simulink model "Task5_without_Scalar"  (R2023b)
settings: Solver=FixedStepAuto  StartTime=0.0  StopTime=500  FixedStep=.02  RelTol=1e-3
values from neighbouring files (symbols this model uses):
  A_Long = [Xu                    Xw                        -w0                            -gravity*cos(theta0) ... (first row only)    [Longitudinal_Autopilot.m]
  B_Long = [Xde                         Xdth ... (first row only)    [Longitudinal_Autopilot.m]
  C_Long = eye(4)    [Longitudinal_Autopilot.m]
  D_Long = zeros(4,2)    [Longitudinal_Autopilot.m]
undefined symbols (not defined in the file or in its folder): states_0, theta0, u0, w0
libraries: simulink_extras x7, cstblocks x2
settings Model: Creator=Saif Mohamed  LastModifiedBy=Saif Mohamed

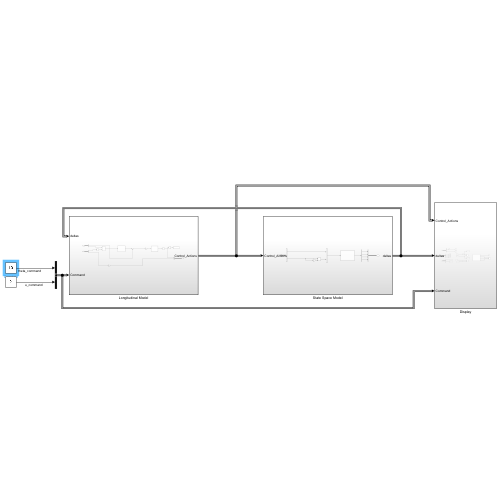
[thumbnail: Simulink's stored preview of the top-level diagram]
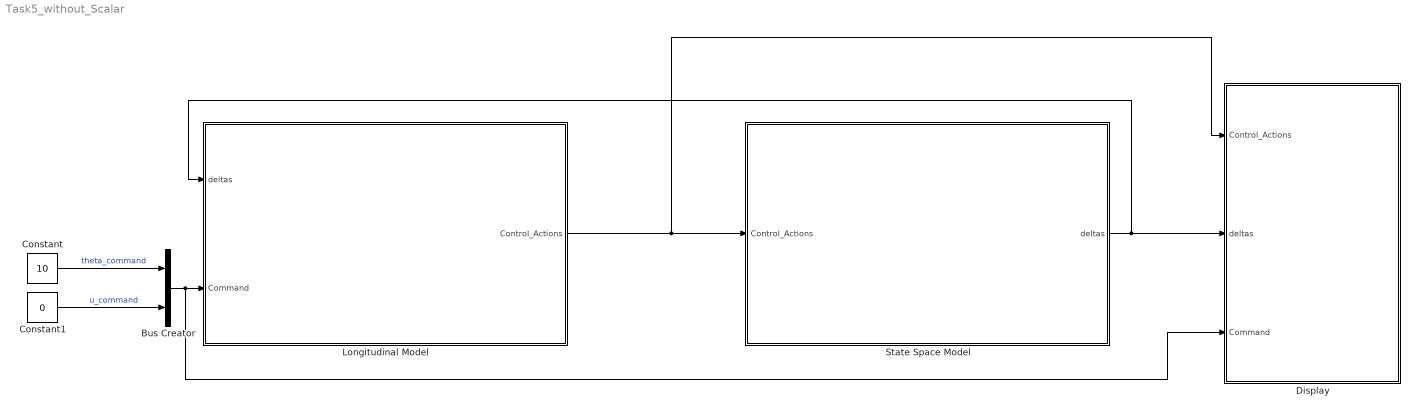
== system Task5_without_Scalar ==
  Bus Creator : BusCreator  Inputs=2
  Constant : Constant  Value=10
  Constant1 : Constant  Value=0
  Display : Subsystem
  Longitudinal Model : Subsystem
  State Space Model : Subsystem
  wires:
  Constant/1 -> Bus Creator/1  "theta_command"
  State Space Model/1(deltas) -> Longitudinal Model/1(deltas), Display/2(deltas)
  Longitudinal Model/1(Control_Actions) -> Display/1(Control_Actions), State Space Model/1(Control_Actions)
  Bus Creator/1 -> Display/3(Command), Longitudinal Model/2(Command)
  Constant1/1 -> Bus Creator/2  "u_command"

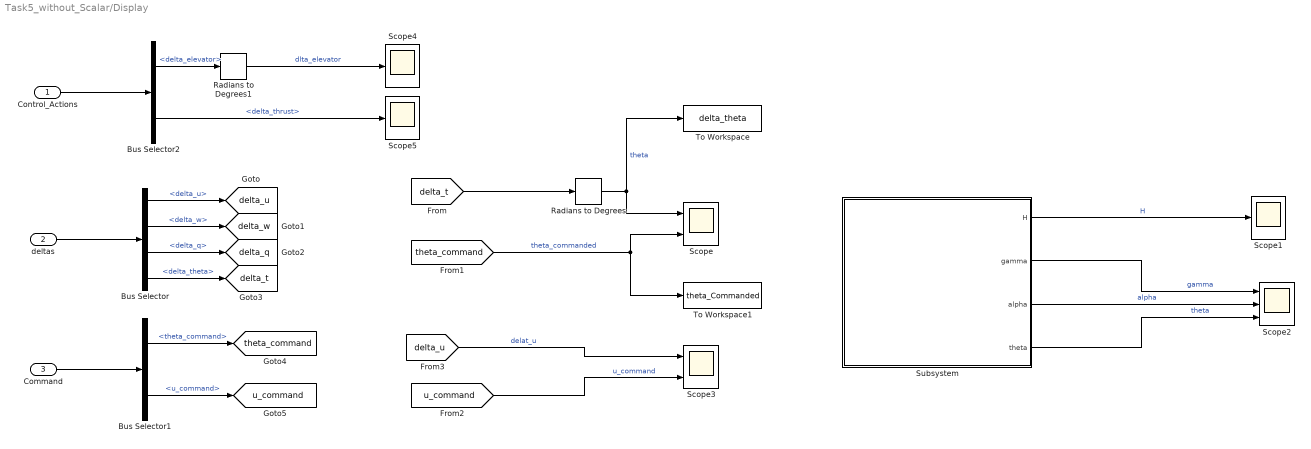
== system Task5_without_Scalar/Display ==
  Control_Actions : Inport
  deltas : Inport  Port=2
  Command : Inport  Port=3
  Bus Selector : BusSelector  OutputSignals=delta_u,delta_w,delta_q,delta_theta
  Bus Selector1 : BusSelector  OutputSignals=theta_command,u_command
  Bus Selector2 : BusSelector  OutputSignals=delta_elevator,delta_thrust
  Radians to Degrees : simulink_extras/Transformations/Radians to Degrees
  Radians to Degrees1 : simulink_extras/Transformations/Radians to Degrees
  Scope : Scope  NumInputPorts=2
  Scope1 : Scope
  Scope2 : Scope  NumInputPorts=3
  Scope3 : Scope  NumInputPorts=2
  Scope4 : Scope
  Scope5 : Scope
  Subsystem : Subsystem
  To Workspace : ToWorkspace  VariableName=delta_theta  SampleTime=-1
  To Workspace1 : ToWorkspace  VariableName=theta_Commanded  SampleTime=-1
  tag scope: delta_q=global, delta_t=global, delta_u=global, delta_w=global, theta_command=global, u_command=global
  wires:
  deltas/1 -> Bus Selector/1
  Bus Selector/1 -> [delta_u]  "<delta_u>"
  Bus Selector/2 -> [delta_w]  "<delta_w>"
  Bus Selector/3 -> [delta_q]  "<delta_q>"
  Bus Selector/4 -> [delta_t]  "<delta_theta>"
  [delta_t] -> Radians to Degrees/1
  Radians to Degrees/1 -> To Workspace/1, Scope/1  "theta"
  [theta_command] -> To Workspace1/1, Scope/2  "theta_commanded"
  Subsystem/1(H) -> Scope1/1  "H"
  Subsystem/3(alpha) -> Scope2/2  "alpha"
  Subsystem/2(gamma) -> Scope2/1  "gamma"
  Subsystem/4(theta) -> Scope2/3  "theta"
  Command/1 -> Bus Selector1/1
  Bus Selector1/1 -> [theta_command]  "<theta_command>"
  Bus Selector1/2 -> [u_command]  "<u_command>"
  [u_command] -> Scope3/2  "u_command"
  [delta_u] -> Scope3/1  "delat_u"
  Control_Actions/1 -> Bus Selector2/1
  Bus Selector2/1 -> Radians to Degrees1/1  "<delta_elevator>"
  Bus Selector2/2 -> Scope5/1  "<delta_thrust>"
  Radians to Degrees1/1 -> Scope4/1  "dlta_elevator"

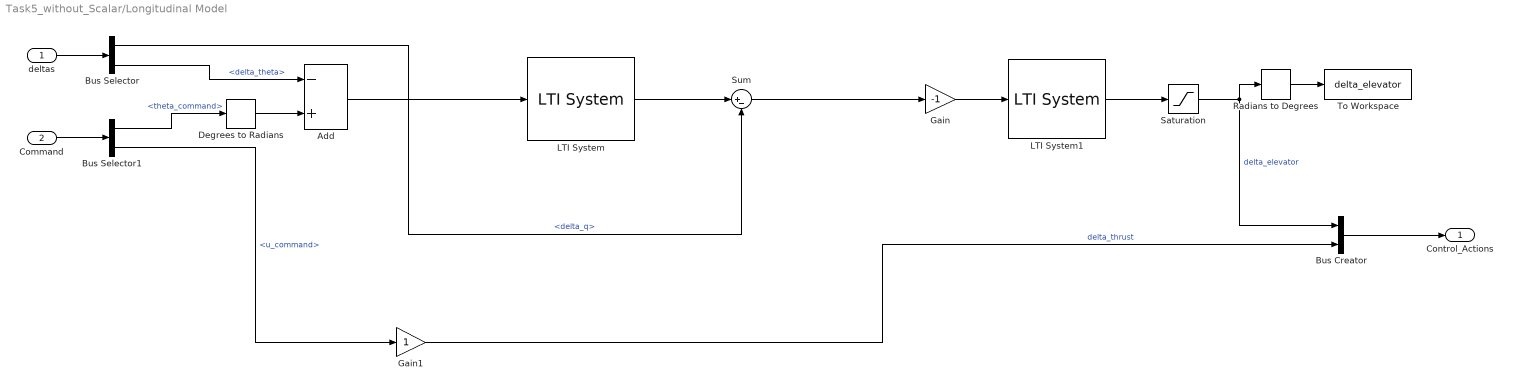
== system Task5_without_Scalar/Longitudinal Model ==
  deltas : Inport
  Command : Inport  Port=2
  Add : Sum  Inputs=-+
  Bus Creator : BusCreator  Inputs=2
  Bus Selector : BusSelector  OutputSignals=delta_q,delta_theta
  Bus Selector1 : BusSelector  OutputSignals=theta_command,u_command
  Degrees to Radians : simulink_extras/Transformations/Degrees to Radians
  Gain : Gain  Gain=-1
  Gain1 : Gain
  LTI System : cstblocks/LTI System  sys=PI_Pitch  IC=[]  PadeOrder=0
  LTI System1 : cstblocks/LTI System  sys=servo  IC=[]  PadeOrder=0
  Radians to Degrees : simulink_extras/Transformations/Radians to Degrees
  Saturation : Saturate  UpperLimit=deg2rad(25)  LowerLimit=deg2rad(-25)
  Sum : Sum  Inputs=|+-
  To Workspace : ToWorkspace  VariableName=delta_elevator  SampleTime=-1
  Control_Actions : Outport
  wires:
  deltas/1 -> Bus Selector/1
  Command/1 -> Bus Selector1/1
  Bus Selector1/1 -> Degrees to Radians/1  "<theta_command>"
  Bus Selector/2 -> Add/1  "<delta_theta>"
  Degrees to Radians/1 -> Add/2
  Add/1 -> LTI System/1
  Bus Selector/1 -> Sum/2  "<delta_q>"
  Sum/1 -> Gain/1
  Gain/1 -> LTI System1/1
  LTI System1/1 -> Saturation/1
  Saturation/1 -> Bus Creator/1, Radians to Degrees/1  "delta_elevator"
  Bus Selector1/2 -> Gain1/1  "<u_command>"
  Gain1/1 -> Bus Creator/2  "delta_thrust"
  Bus Creator/1 -> Control_Actions/1
  Radians to Degrees/1 -> To Workspace/1
  LTI System/1 -> Sum/1

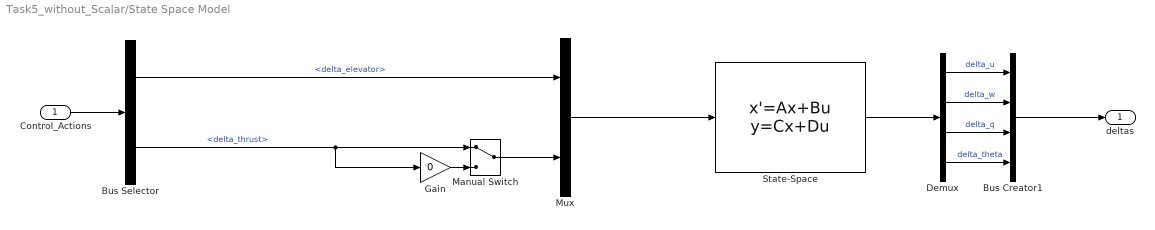
== system Task5_without_Scalar/State Space Model ==
  Control_Actions : Inport
  Bus Creator1 : BusCreator  Inputs=4
  Bus Selector : BusSelector  OutputSignals=delta_elevator,delta_thrust
  Demux : Demux
  Gain : Gain  Gain=0
  Manual Switch : ManualSwitch
  Mux : Mux  Inputs=2
  State-Space : StateSpace  A=A_Long  B=B_Long  C=C_Long  D=D_Long  InitialCondition=0
  deltas : Outport
  wires:
  Demux/3 -> Bus Creator1/3  "delta_q"
  Mux/1 -> State-Space/1
  Demux/2 -> Bus Creator1/2  "delta_w"
  Demux/1 -> Bus Creator1/1  "delta_u"
  Bus Creator1/1 -> deltas/1
  State-Space/1 -> Demux/1
  Demux/4 -> Bus Creator1/4  "delta_theta"
  Manual Switch/1 -> Mux/2
  Gain/1 -> Manual Switch/2
  Control_Actions/1 -> Bus Selector/1
  Bus Selector/1 -> Mux/1  "<delta_elevator>"
  Bus Selector/2 -> Gain/1, Manual Switch/1  "<delta_thrust>"

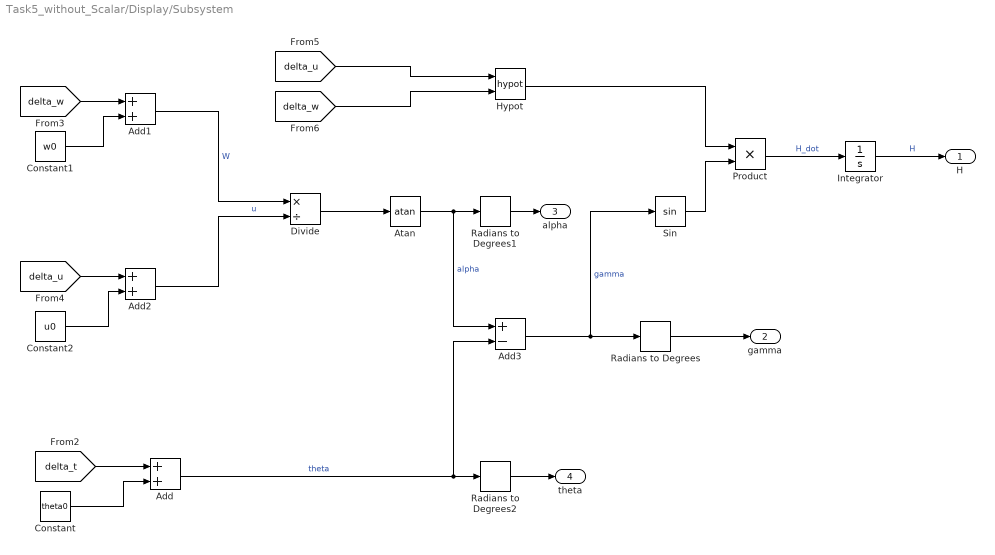
== system Task5_without_Scalar/Display/Subsystem ==
  Add : Sum
  Add1 : Sum
  Add2 : Sum
  Add3 : Sum  Inputs=+-
  Atan : Trigonometry  Operator=atan
  Constant : Constant  Value=theta0
  Constant1 : Constant  Value=w0
  Constant2 : Constant  Value=u0
  Divide : Product  Inputs=*/
  Hypot : Math  Operator=hypot
  Integrator : Integrator  InitialCondition=-states_0(12)
  Product : Product
  Radians to Degrees : simulink_extras/Transformations/Radians to Degrees
  Radians to Degrees1 : simulink_extras/Transformations/Radians to Degrees
  Radians to Degrees2 : simulink_extras/Transformations/Radians to Degrees
  Sin : Trigonometry
  H : Outport
  gamma : Outport  Port=2
  alpha : Outport  Port=3
  theta : Outport  Port=4
  wires:
  [delta_w] -> Hypot/2
  Integrator/1 -> H/1  "H"
  [delta_t] -> Add/1
  Add/1 -> Radians to Degrees2/1, Add3/2  "theta"
  [delta_u] -> Hypot/1
  Constant1/1 -> Add1/2
  Sin/1 -> Product/2
  [delta_u] -> Add2/1
  [delta_w] -> Add1/1
  Constant2/1 -> Add2/2
  Constant/1 -> Add/2
  Add3/1 -> Radians to Degrees/1, Sin/1  "gamma"
  Product/1 -> Integrator/1  "H_dot"
  Add2/1 -> Divide/2  "u"
  Atan/1 -> Add3/1, Radians to Degrees1/1  "alpha"
  Hypot/1 -> Product/1
  Divide/1 -> Atan/1
  Add1/1 -> Divide/1  "W"
  Radians to Degrees/1 -> gamma/1
  Radians to Degrees1/1 -> alpha/1
  Radians to Degrees2/1 -> theta/1
